simulink model "gm_delay"  (R2018a)
settings: Solver=VariableStepAuto  StartTime=0.0  StopTime=10.0  RelTol=1e-3
libraries: dspvision x2
settings Model: Creator=Lu  LastModifiedBy=Lu
settings OptimizationCC: BlockReduction=off  ConditionallyExecuteInputs=off
settings DebuggingCC: InheritedTsInSrcMsg=none

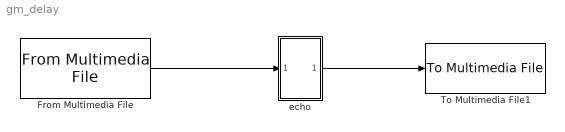
== system gm_delay ==
  From Multimedia File : dspvision/From Multimedia File  inputFilename=C:\Users\lugfe\Documents\GitHub\dsp-fpgay\TP FINAL\audio effects\little-wing.wav  loop=on  numPlays=1  outputStreams=Audio only  videoDataType=single  audioDataType=int16  inheritSampleTime=on  userDefinedSampleTime=1/30  noAudioOutput=off  isIntensityVideo=off  fourcc=RGB  colorVideoFormat=Separate color signals  outputEOF=off  dataOrg=Column-major  audioFrameSize=1  computeAudioFrameSize=off  outSamplingMode=Sample based
      settings: SourceProductBaseCode=VP
  To Multimedia File1 : dspvision/To Multimedia File  outputFilename=C:\Users\lugfe\Documents\GitHub\dsp-fpgay\TP FINAL\audio effects\delay_little-wing.wav  streamSelection=Audio only  videoCompressor=None (uncompressed)  audioCompressor=None (uncompressed)  imagePorts=Separate color signals  fileType=WAV  audioDatatype=Determine from input data type  fourcc=RGB  videoQuality=75  mj2000CompFactor=10
      settings: SourceProductName=Computer Vision System Toolbox  SourceProductBaseCode=VP
  echo : Subsystem
  wires:
  echo/1(Out1) -> To Multimedia File1/1
  From Multimedia File/1 -> echo/1(In1)

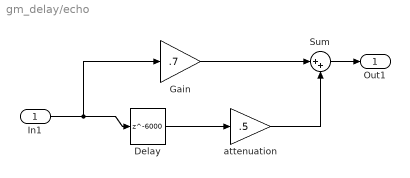
== system gm_delay/echo ==
  In1 : Inport  OutDataTypeStr=int16
  Delay : Delay  DelayLength=6000  DelayLengthUpperLimit=10000  InitialCondition=0  InputProcessing=Columns as channels (frame based)
  Gain : Gain  Gain=.7  ParamDataTypeStr=int16  OutDataTypeStr=int16
  Sum : Sum  Inputs=|++
  attenuation : Gain  Gain=.5  OutDataTypeStr=int16  RndMeth=Round
  Out1 : Outport
  wires:
  Delay/1 -> attenuation/1
  Sum/1 -> Out1/1
  Gain/1 -> Sum/1
  attenuation/1 -> Sum/2
  In1/1 -> Gain/1, Delay/1
